simulink model "Resp18e_updatedPulse"  (Simulink 7.3)
settings: Solver=ode23  StartTime=0.0  StopTime=20  FixedStep=0.01  MaxStep=0.05  RelTol=1e-6
values from neighbouring files (symbols this model uses):
  alpha_CO2_brain = 2.9/1e3*760/P_stp/K_stp    (= 0.00097047576489)    [initialize_parameters.m]
  alpha_CO2_fat = 0.9/K_stp/P_stp    (= 0.000396292281489)    [initialize_parameters.m]
  alpha_CO2_heart = 2.4/1e3*760/P_stp/K_stp    (= 0.00080315235715)    [initialize_parameters.m]
  alpha_CO2_lean = 4.2/1e3*760/P_stp/K_stp    (= 0.00140551662501)    [initialize_parameters.m]
  alpha_CO2_lungtiss_fast = alpha_CO2_lungtiss_fast./0.1333    [initialize_parameters.m]
  alpha_CO2_muscle = 4.2/1e3*760/P_stp/K_stp    (= 0.00140551662501)    [initialize_parameters.m]
  alpha_CO2_other = 3.0/1e3*760/P_stp/K_stp    (= 0.00100394044644)    [initialize_parameters.m]
  alpha_O2_fat = 5*0.024/K_stp/P_stp    (= 5.28389708651e-05)    [initialize_parameters.m]
  alpha_O2_tissue = 0.024/K_stp/P_stp    (= 1.0567794173e-05)    [initialize_parameters.m]
  BOHRF0 = O2_SHIFT - T_BLOOD_M_37 * (0.024 + BOHRF * 0.0147) - BOHRF1 * 7.4    (= -3.552)    [initialize_parameters.m]
  BOHRF1 = BOHRF * (1 - T_BLOOD_M_37 * 0.0065)    (= 0.48)    [initialize_parameters.m]
  C_a_CO2_i = 20.8e-3    (= 0.0208)    [initialize_parameters.m]    (also in resp18e_ic_norm.mat = 0.0202734801806)
  C_a_O2_i = 8.95e-3    (= 0.00895)    [initialize_parameters.m]    (also in resp18e_ic_norm.mat = 0.00918087581167)
  CAP_O2 = 0.01 * CAP_O2    (= 0.201)    [initialize_parameters.m]
  Cardiac_duty_cycle = 40    [initialize_parameters.m]
  Co_CO2_brain = 401*K_Co_CO2/1e3/K_stp    (= 0.0107345869894)    [initialize_parameters.m]
  Co_CO2_heart = 487*K_Co_CO2/1e3/K_stp    (= 0.0130367677403)    [initialize_parameters.m]
  Co_CO2_lean = 342*K_Co_CO2/1e3/K_stp    (= 0.00915518391618)    [initialize_parameters.m]
  Co_CO2_muscle = 342*K_Co_CO2/1e3/K_stp    (= 0.00915518391618)    [initialize_parameters.m]
  Co_CO2_other = 355*K_Co_CO2/1e3/K_stp    (= 0.00950318798317)    [initialize_parameters.m]
  DH2ODS = DH2ODS + 0.007 * HB_MEQ * (HB_MEQ - 9) / (13.5 * (13.5 - 9))    (= 0.00498709726946)    [initialize_parameters.m]
  F_insp_alv_alvds = F_v_alv_deadspace / F_insp_hivq    (= 0.00299401197605)    [initialize_parameters.m]
  F_insp_alv_hivq = F_v_alv_hivq      / F_insp_hivq    (= 0.997005988024)    [initialize_parameters.m]
  F_insp_alv_lovq = F_v_alv_lovq      / F_insp_lovq    (= 0.5)    [initialize_parameters.m]
  F_insp_alv_midvq = F_v_alv_midvq     / F_insp_lovq    (= 0.5)    [initialize_parameters.m]
  F_insp_hivq = F_v_alv_deadspace + F_v_alv_hivq    (= 0.334)    [initialize_parameters.m]
  F_insp_lovq = F_v_alv_midvq     + F_v_alv_lovq    (= 0.666)    [initialize_parameters.m]
  Fi_CO2_param_est = 0.01    [initialize_parameters.m]
  Fi_error = 1e-6    (= 1e-06)    [initialize_parameters.m]
  Fi_N2_mean = 1-(Fi_O2_mean + Fi_N2O_mean)    (= 0.65)    [initialize_parameters.m]
  Fi_O2_mean = 0.35    [initialize_parameters.m]
  Fi_O2_param_est = 0.01    [initialize_parameters.m]
  Fq_brain = 0.114    [initialize_parameters.m]
  Fq_error = 1e-8    (= 1e-08)    [initialize_parameters.m]
  Fq_fat = 0.103    [initialize_parameters.m]
  Fq_heart = 0.041    [initialize_parameters.m]
  Fq_hepatic = 0.069    [initialize_parameters.m]
  Fq_kidneys = 0.215    [initialize_parameters.m]
  Fq_lean = 0.090    (= 0.09)    [initialize_parameters.m]
  Fq_lungs_anatomicalshunt = 0.01    [initialize_parameters.m]
  Fq_lungs_hivq = (1-Fq_lungs_pulmshunt-Fq_lungs_anatomicalshunt)    *F_v_alv_hivq/(F_v_alv_hivq+F_v_alv_midvq+F_v_alv_lovq)    (= 0.3)    [initialize_parameters.m]
  Fq_lungs_lovq = (1-Fq_lungs_pulmshunt-Fq_lungs_anatomicalshunt)    *F_v_alv_lovq/(F_v_alv_hivq+F_v_alv_midvq+F_v_alv_lovq)    (= 0.3)    [initialize_parameters.m]
  Fq_lungs_midvq = (1-Fq_lungs_pulmshunt-Fq_lungs_anatomicalshunt)    *F_v_alv_midvq/(F_v_alv_hivq+F_v_alv_midvq+F_v_alv_lovq)    (= 0.3)    [initialize_parameters.m]
  Fq_lungs_pulmshunt = 0.09    [initialize_parameters.m]
  Fq_muscle = 0.096    [initialize_parameters.m]
  Fq_pershunt = 0.101    [initialize_parameters.m]
  Fq_portal = 0.171    [initialize_parameters.m]
  FRC = 2.2    [initialize_parameters.m]
  H2OB = H2OVC + 0.938 * (1 - VC_74)    (= 0.840191964286)    [initialize_parameters.m]
  k_CO2_lungtiss_fast_alvds = k_CO2_lungtiss_fast*F_v_alv_deadspace    (= 3.63090772693e-07)    [initialize_parameters.m]
  k_CO2_lungtiss_fast_hivq = k_CO2_lungtiss_fast*F_v_alv_hivq    (= 0.000120909227307)    [initialize_parameters.m]
  k_CO2_lungtiss_fast_lovq = k_CO2_lungtiss_fast*F_v_alv_lovq    (= 0.000120909227307)    [initialize_parameters.m]
  k_CO2_lungtiss_fast_midvq = k_CO2_lungtiss_fast*F_v_alv_midvq    (= 0.000120909227307)    [initialize_parameters.m]
  k_CO2_lungtiss_slow_alvds = k_CO2_lungtiss_slow*F_v_alv_deadspace    (= 4.95123780945e-09)    [initialize_parameters.m]
  k_CO2_lungtiss_slow_hivq = k_CO2_lungtiss_slow*F_v_alv_hivq    (= 1.64876219055e-06)    [initialize_parameters.m]
  k_CO2_lungtiss_slow_lovq = k_CO2_lungtiss_slow*F_v_alv_lovq    (= 1.64876219055e-06)    [initialize_parameters.m]
  k_CO2_lungtiss_slow_midvq = k_CO2_lungtiss_slow*F_v_alv_midvq    (= 1.64876219055e-06)    [initialize_parameters.m]
  K_diff_CO2_hivq = K_diff_CO2*F_v_alv_hivq    (= 0.0014985)    [initialize_parameters.m]
  K_diff_CO2_lovq = K_diff_CO2*F_v_alv_lovq    (= 0.0014985)    [initialize_parameters.m]
  K_diff_CO2_midvq = K_diff_CO2*F_v_alv_midvq    (= 0.0014985)    [initialize_parameters.m]
  K_diff_O2_hivq = K_diff_O2*F_v_alv_hivq    (= 7.326e-05)    [initialize_parameters.m]
  K_diff_O2_lovq = K_diff_O2*F_v_alv_lovq    (= 7.326e-05)    [initialize_parameters.m]
  K_diff_O2_midvq = K_diff_O2*F_v_alv_midvq    (= 7.326e-05)    [initialize_parameters.m]
  K_exp_alv_alvds = 1/1    (= 1)    [initialize_parameters.m]
  K_exp_alv_hivq = 1/1    (= 1)    [initialize_parameters.m]
  K_press = 760/101.325    (= 7.50061682704)    [initialize_parameters.m]
  K_stp = R*(T_stp+273.15)/(P_stp*1000)    (= 22.4135311621)    [initialize_parameters.m]
  Kg_alv = R*(T_alv+273.15)/(P_baro*1000)    (= 25.3668469802)    [initialize_parameters.m]
  LN10 = 2.30258509299405    (= 2.30258509299)    [initialize_parameters.m]
  m_alv_alvds_i = (FRC-V_deadspace_total)/Kg_alv * F_v_alv_deadspace    [initialize_parameters.m]
  m_alv_hivq_i = (FRC-V_deadspace_total)/Kg_alv * F_v_alv_hivq    [initialize_parameters.m]
  m_alv_lovq_i = (FRC-V_deadspace_total)/Kg_alv * F_v_alv_lovq    [initialize_parameters.m]
  m_alv_midvq_i = (FRC-V_deadspace_total)/Kg_alv * F_v_alv_midvq    [initialize_parameters.m]
  m_CO2_alv_alvds_i = F_CO2_i * m_alv_alvds_i    [initialize_parameters.m]
  m_CO2_alv_hivq_i = F_CO2_i * m_alv_hivq_i    [initialize_parameters.m]
  m_CO2_alv_lovq_i = F_CO2_i * m_alv_lovq_i    [initialize_parameters.m]
  m_CO2_alv_midvq_i = F_CO2_i * m_alv_midvq_i    [initialize_parameters.m]
  m_CO2_brain_b_i = C_a_CO2_i*Vb_brain    (= 0.002184)    [initialize_parameters.m]
  m_CO2_brain_t_i = (Co_CO2_brain  + alpha_CO2_brain *P_v_CO2_i)* Vt_brain    (= 0.0171268217946)    [initialize_parameters.m]
  m_CO2_common_b_i = C_a_CO2_i*Vb_common    (= 0.0170421333333)    [initialize_parameters.m]
  m_CO2_ds0_i = F_CO2_i*m_ds0_i    (= 0.000985538329597)    [initialize_parameters.m]
  m_CO2_ds_large_i = F_CO2_i * m_deadspace_large_1    [initialize_parameters.m]
  m_CO2_ds_med_hivq1_i = F_CO2_i * m_deadspace_med_hivq_1    [initialize_parameters.m]
  m_CO2_ds_med_hivq2_i = F_CO2_i * m_deadspace_med_hivq_2    [initialize_parameters.m]
  m_CO2_ds_med_lovq1_i = F_CO2_i * m_deadspace_med_lovq_1    [initialize_parameters.m]
  m_CO2_ds_med_lovq2_i = F_CO2_i * m_deadspace_med_lovq_2    [initialize_parameters.m]
  m_CO2_ds_small_alvds_i = F_CO2_i * m_deadspace_small_alvdeadspace    [initialize_parameters.m]
  m_CO2_ds_small_hivq_i = F_CO2_i * m_deadspace_small_hivq    [initialize_parameters.m]
  m_CO2_ds_small_lovq_i = F_CO2_i * m_deadspace_small_lovq    [initialize_parameters.m]
  m_CO2_ds_small_midvq_i = F_CO2_i * m_deadspace_small_midvq    [initialize_parameters.m]
  m_CO2_fat_b_i = C_a_CO2_i*Vb_fat    (= 0.0116896)    [initialize_parameters.m]
  m_CO2_fat_t_i = P_a_CO2_i*alpha_CO2_fat*Vt_fat    (= 0.0302752719501)    [initialize_parameters.m]
  m_CO2_heart_b_i = C_a_CO2_i*Vb_heart    (= 0.000832)    [initialize_parameters.m]
  m_CO2_heart_t_i = (Co_CO2_heart  + alpha_CO2_heart *P_v_CO2_i)* Vt_heart    (= 0.00402544335149)    [initialize_parameters.m]
  m_CO2_hepatic_b_i = C_a_CO2_i*Vb_hepatic    (= 0.0019136)    [initialize_parameters.m]
  m_CO2_kidneys_b_i = C_a_CO2_i*Vb_kidneys    (= 0.0012064)    [initialize_parameters.m]
  m_CO2_kidneys_t_i = (Co_CO2_other  + alpha_CO2_other *P_v_CO2_i)* Vt_kidneys    (= 0.0045902552907)    [initialize_parameters.m]
  m_CO2_lean_b_i = C_a_CO2_i*Vb_lean    (= 0.0191984)    [initialize_parameters.m]
  m_CO2_lean_t_i = (Co_CO2_lean   + alpha_CO2_lean  *P_v_CO2_i)* Vt_lean    (= 0.0884995401953)    [initialize_parameters.m]
  m_CO2_liver_t_i = (Co_CO2_other  + alpha_CO2_other *P_v_CO2_i)* Vt_liver    (= 0.0187019339777)    [initialize_parameters.m]
  m_CO2_lungtiss_fast_alvds_i = F_CO2_i*(P_baro-P_A_H2O)*V_lungtiss_alvds *alpha_CO2_lungtiss_fast(2)    [initialize_parameters.m]
  m_CO2_lungtiss_fast_hivq_i = F_CO2_i*(P_baro-P_A_H2O)*V_lungtiss_hivq  *alpha_CO2_lungtiss_fast(2)    [initialize_parameters.m]
  m_CO2_lungtiss_fast_lovq_i = F_CO2_i*(P_baro-P_A_H2O)*V_lungtiss_lovq  *alpha_CO2_lungtiss_fast(2)    [initialize_parameters.m]
  m_CO2_lungtiss_fast_midvq_i = F_CO2_i*(P_baro-P_A_H2O)*V_lungtiss_midvq *alpha_CO2_lungtiss_fast(2)    [initialize_parameters.m]
  m_CO2_lungtiss_slow_alvds_i = F_CO2_i*(P_baro-P_A_H2O)*V_lungtiss_alvds*alpha_CO2_lungtiss_slow    [initialize_parameters.m]
  m_CO2_lungtiss_slow_hivq_i = F_CO2_i*(P_baro-P_A_H2O)*V_lungtiss_hivq *alpha_CO2_lungtiss_slow    [initialize_parameters.m]
  m_CO2_lungtiss_slow_lovq_i = F_CO2_i*(P_baro-P_A_H2O)*V_lungtiss_lovq *alpha_CO2_lungtiss_slow    [initialize_parameters.m]
  m_CO2_lungtiss_slow_midvq_i = F_CO2_i*(P_baro-P_A_H2O)*V_lungtiss_midvq*alpha_CO2_lungtiss_slow    [initialize_parameters.m]
  m_CO2_LV_b_i = C_a_CO2_i*Vb_LV    (= 0.00391733333333)    [initialize_parameters.m]
  m_CO2_muscle_b_i = C_a_CO2_i*Vb_muscle    (= 0.0201344)    [initialize_parameters.m]
  m_CO2_muscle_t_i = (Co_CO2_muscle + alpha_CO2_muscle*P_v_CO2_i)* Vt_muscle    (= 0.363660431061)    [initialize_parameters.m]
  m_CO2_pershunt_b_i = C_a_CO2_i*Vb_pershunt    (= 0.0027248)    [initialize_parameters.m]
  m_CO2_portal_b_i = C_a_CO2_i*Vb_portal    (= 0.0210912)    [initialize_parameters.m]
  m_CO2_portal_t_i = (Co_CO2_other  + alpha_CO2_other *P_v_CO2_i)* Vt_portal    (= 0.0164739329706)    [initialize_parameters.m]
  m_CO2_pulmcap_b_hivq_i = C_a_CO2_i*Vb_pulmcap_hivq    (= 0.000630933333333)    [initialize_parameters.m]
  m_CO2_pulmcap_b_lovq_i = C_a_CO2_i*Vb_pulmcap_lovq    (= 0.000630933333333)    [initialize_parameters.m]
  m_CO2_pulmcap_b_midvq_i = C_a_CO2_i*Vb_pulmcap_midvq    (= 0.000630933333333)    [initialize_parameters.m]
  m_CO2_pulmcap_b_pulmshunt_i = C_a_CO2_i*Vb_pulmcap_pulmshunt    (= 0.0001872)    [initialize_parameters.m]
  m_CO2_RV_b_i = C_v_CO2_i*Vb_RV    (= 0.004181)    [initialize_parameters.m]
  m_N2_alv_alvds_i = Fi_N2_mean * (m_alv_alvds_i - m_CO2_alv_alvds_i)    [initialize_parameters.m]
  ... (+122 more)
undefined symbols (not defined in the file or in its folder): AH2OVC, AHCO3B, DHCO3BDS, litres, mole
libraries: simulink x28
(part 1 of 8)
settings Model: Creator=MJTurner  LastModifiedBy=John  ExtModeTrigMode=oneshot  ExtModeArmWhenConnect=off
settings SolverCC: InitialStep=0.0001  MaxOrder=3
settings DataIOCC: FinalStateName=x_final  InitialState=x_initial  LimitDataPoints=off  LoadInitialState=on  SaveFinalState=on  SaveOutput=off  StateSaveName=x_states  TimeSaveName=t
settings OptimizationCC: BlockReduction=off  BooleanDataType=off  InitFltsAndDblsToZero=on
settings DebuggingCC: AlgebraicLoopMsg=none  SaveWithParameterizedLinksMsg=none  SignalResolutionControl=TryResolveAllWithWarning  SolverPrmCheckMsg=none  MultiTaskDSMMsg=warning  MultiTaskCondExecSysMsg=none  StrictBusMsg=None
settings HardwareCC: TargetUnknown=on
settings RTWCC: TemplateMakefile=grt_vc.tmf  IncludeERTFirstTime=on
settings GRTTargetCC: TargetFcnLib=ansi_tfl_tmw.mat

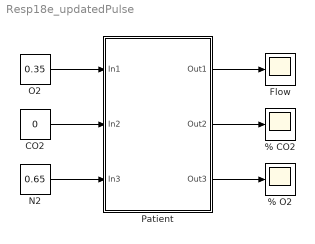
== system Resp18e_updatedPulse ==
  % CO2 : Scope
      settings: YMin=0  YMax=5.25  SaveName=ScopeData9
  % O2 : Scope
      settings: YMin=28.5  YMax=35  SaveName=ScopeData8
  CO2 : Constant  Value=0  OutDataType=fixdt(1, 16)  OutScaling=2^0
  Flow : Scope
      settings: YMin=-0.02  YMax=0.0175  SaveName=ScopeData10
  N2 : Constant  Value=0.65  OutDataType=fixdt(1, 16)  OutScaling=2^0
  O2 : Constant  Value=0.35  OutDataType=fixdt(1, 16)  OutScaling=2^0
  Patient : Subsystem
  wires:
  O2/1 -> Patient/1(In1)
  CO2/1 -> Patient/2(In2)
  N2/1 -> Patient/3(In3)
  Patient/3(Out3) -> % O2/1
  Patient/1(Out1) -> Flow/1
  Patient/2(Out2) -> % CO2/1

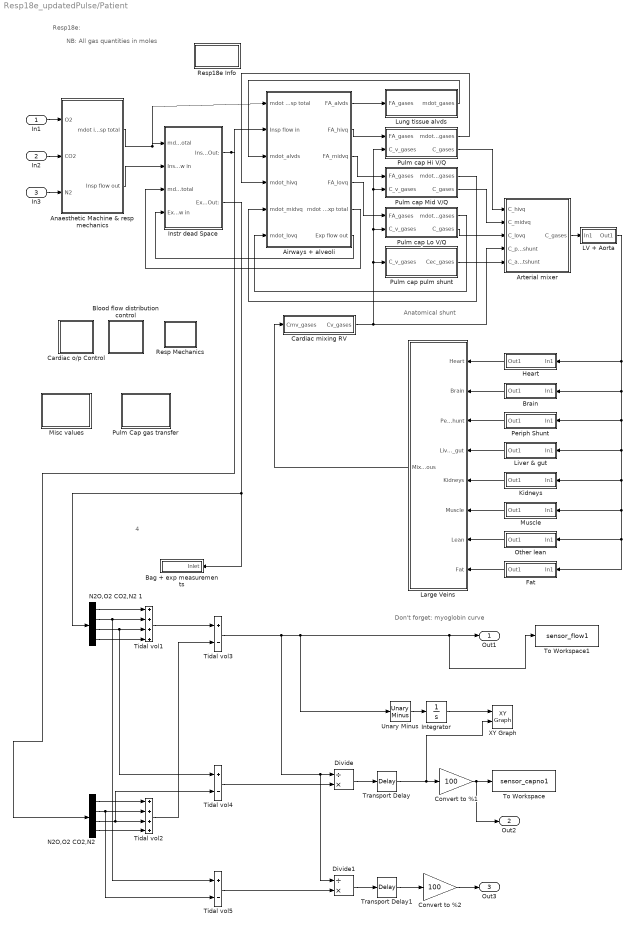
== system Resp18e_updatedPulse/Patient ==
  note: Resp18e:
  note: NB: All gas quantities in moles
  note: Anatomical shunt
  note: 4
  note: Don't forget: myoglobin curve
  In1 : Inport
  In2 : Inport  Port=2
  In3 : Inport  Port=3
  Airways + alveoli : Subsystem
  Anaesthetic Machine & resp mechanics : Subsystem
  Arterial mixer : Subsystem
  Bag + exp measurements : Subsystem
  Blood flow distribution control : Subsystem
  Brain : Subsystem
  Cardiac mixing RV : Subsystem
  Cardiac o/p Control : Subsystem
  Convert to %1 : Gain  Gain=100  ParameterDataType=fixdt(1, 16)  ParameterScaling=2^0  OutDataType=fixdt(1, 16)  OutScaling=2^0
  Convert to %2 : Gain  Gain=100  ParameterDataType=fixdt(1, 16)  ParameterScaling=2^0  OutDataType=fixdt(1, 16)  OutScaling=2^0
  Divide : Product  Inputs=/*  OutDataType=fixdt(1, 16)  OutScaling=2^-10
  Divide1 : Product  Inputs=/*  OutDataType=fixdt(1, 16)  OutScaling=2^-10
  Fat : Subsystem
  Heart : Subsystem
  Instr dead Space : Subsystem
  Integrator : Integrator  ZeroCross=off  ContinuousStateAttributes='volumeIntegrator'
  Kidneys : Subsystem
  LV + Aorta : Subsystem
  Large Veins : Subsystem
  Liver & gut : Subsystem
  Lung tissue alvds : Subsystem
  Misc values : Subsystem
  Muscle : Subsystem
  "N2O,O2 CO2,N2 " : Demux
  N2O,O2 CO2,N2 1 : Demux
  Other lean : Subsystem
  Periph Shunt : Subsystem
  Pulm Cap gas transfer : Subsystem
  Pulm cap Hi V/Q : Subsystem
  Pulm cap Lo V/Q : Subsystem
  Pulm cap Mid V/Q : Subsystem
  Pulm cap pulm shunt : Subsystem
  Resp Mechanics : Subsystem
  Resp18e Info : Subsystem
  Tidal vol1 : Sum  Inputs=++++  OutDataType=sfix(16)  OutScaling=2^0  SaturateOnIntegerOverflow=on  InputSameDT=on  OutDataTypeStr=Inherit: Same as first input
  Tidal vol2 : Sum  Inputs=++++  OutDataType=sfix(16)  OutScaling=2^0  SaturateOnIntegerOverflow=on  InputSameDT=on  OutDataTypeStr=Inherit: Same as first input
  Tidal vol3 : Sum  Inputs=+-  OutDataType=sfix(16)  OutScaling=2^0  SaturateOnIntegerOverflow=on  InputSameDT=on  OutDataTypeStr=Inherit: Same as first input
  Tidal vol4 : Sum  Inputs=+-  OutDataType=sfix(16)  OutScaling=2^0  SaturateOnIntegerOverflow=on  InputSameDT=on  OutDataTypeStr=Inherit: Same as first input
  Tidal vol5 : Sum  Inputs=+-  OutDataType=sfix(16)  OutScaling=2^0  SaturateOnIntegerOverflow=on  InputSameDT=on  OutDataTypeStr=Inherit: Same as first input
  To Workspace : ToWorkspace  VariableName=sensor_capno1  SampleTime=t_sample_sensor  SaveFormat=Array
  To Workspace1 : ToWorkspace  VariableName=sensor_flow1  SampleTime=t_sample_sensor  SaveFormat=Array
  Transport Delay : TransportDelay  DelayTime=0.01
  Transport Delay1 : TransportDelay  DelayTime=0.01
  Unary Minus : simulink/Math Operations/Unary Minus  DoSatur=off
  XY Graph : simulink/Sinks/XY Graph  SystemSampleTime=-1  xmin=-0.05  xmax=0.05  ymin=0  ymax=0.08  st=-1
  Out1 : Outport
  Out2 : Outport  Port=2
  Out3 : Outport  Port=3
  wires:
  Anaesthetic Machine & resp mechanics/2(Insp flow out) -> Instr dead Space/2(Insp flow in)
  Instr dead Space/2(Exp flow Out:) -> Bag + exp measurements/1(Inlet), N2O,O2 CO2,N2 1/1
  Anaesthetic Machine & resp mechanics/1(mdot insp total) -> Instr dead Space/1(mdot InspTotal), Airways + alveoli/1(mdot insp total)
  Instr dead Space/1(Insp flow Out:) -> Airways + alveoli/2(Insp flow in), "N2O,O2 CO2,N2 "/1
  Airways + alveoli/6(Exp flow out) -> Instr dead Space/4(Exp flow in)
  Arterial mixer/1(C_gases) -> LV + Aorta/1(In1)
  Airways + alveoli/2(FA_hivq) -> Pulm cap Hi V/Q/1(FA_gases)
  Airways + alveoli/3(FA_midvq) -> Pulm cap Mid V/Q/1(FA_gases)
  Airways + alveoli/4(FA_lovq) -> Pulm cap Lo V/Q/1(FA_gases)
  Pulm cap Lo V/Q/1(mdot_gases) -> Airways + alveoli/6(mdot_lovq)
  Pulm cap Mid V/Q/1(mdot_gases) -> Airways + alveoli/5(mdot_midvq)
  Pulm cap Hi V/Q/1(mdot_gases) -> Airways + alveoli/4(mdot_hivq)
  Pulm cap Lo V/Q/2(C_gases) -> Arterial mixer/3(C_lovq)
  Pulm cap Mid V/Q/2(C_gases) -> Arterial mixer/2(C_midvq)
  Pulm cap Hi V/Q/2(C_gases) -> Arterial mixer/1(C_hivq)
  Lung tissue alvds/1(mdot_gases) -> Airways + alveoli/3(mdot_alvds)
  Airways + alveoli/1(FA_alvds) -> Lung tissue alvds/1(FA_gases)
  Liver & gut/1(Out1) -> Large Veins/4(Liver_gut)
  LV + Aorta/1(Out1) -> Heart/1(In1), Liver & gut/1(In1), Kidneys/1(In1), Muscle/1(In1), Other lean/1(In1), Fat/1(In1), Periph Shunt/1(In1), Brain/1(In1)
  Heart/1(Out1) -> Large Veins/1(Heart)
  Kidneys/1(Out1) -> Large Veins/5(Kidneys)
  Muscle/1(Out1) -> Large Veins/6(Muscle)
  Other lean/1(Out1) -> Large Veins/7(Lean)
  Fat/1(Out1) -> Large Veins/8(Fat)
  Brain/1(Out1) -> Large Veins/2(Brain)
  Periph Shunt/1(Out1) -> Large Veins/3(Per shunt)
  Cardiac mixing RV/1(Cv_gases) -> Arterial mixer/4(C_pulmshunt), Pulm cap Lo V/Q/2(C_v_gases), Pulm cap Mid V/Q/2(C_v_gases), Pulm cap Hi V/Q/2(C_v_gases), Pulm cap pulm shunt/1(C_v_gases)
  Large Veins/1(Mixed Venous) -> Cardiac mixing RV/1(Cmv_gases)
  Pulm cap pulm shunt/1(Cec_gases) -> Arterial mixer/5(C_anatshunt)
  Airways + alveoli/5(mdot exp total) -> Instr dead Space/3(mdot exp total)
  N2O,O2 CO2,N2 1/1 -> Tidal vol1/1
  N2O,O2 CO2,N2 1/4 -> Tidal vol1/4
  N2O,O2 CO2,N2 1/2 -> Tidal vol1/2, Tidal vol5/1
  "N2O,O2 CO2,N2 "/1 -> Tidal vol2/1
  "N2O,O2 CO2,N2 "/2 -> Tidal vol2/2, Tidal vol5/2
  Tidal vol1/1 -> Tidal vol3/1
  N2O,O2 CO2,N2 1/3 -> Tidal vol1/3, Tidal vol4/1
  "N2O,O2 CO2,N2 "/3 -> Tidal vol2/3, Tidal vol4/2
  "N2O,O2 CO2,N2 "/4 -> Tidal vol2/4
  Tidal vol2/1 -> Tidal vol3/2
  Tidal vol4/1 -> Divide/2
  Tidal vol3/1 -> Unary Minus/1, To Workspace1/1, Out1/1, Divide/1, Divide1/1
  Divide/1 -> Transport Delay/1
  Transport Delay/1 -> XY Graph/2, Convert to %1/1
  Integrator/1 -> XY Graph/1
  Unary Minus/1 -> Integrator/1
  Divide1/1 -> Transport Delay1/1
  Tidal vol5/1 -> Divide1/2
  In1/1 -> Anaesthetic Machine & resp mechanics/1(O2)
  In2/1 -> Anaesthetic Machine & resp mechanics/2(CO2)
  In3/1 -> Anaesthetic Machine & resp mechanics/3(N2)
  Transport Delay1/1 -> Convert to %2/1
  Convert to %1/1 -> To Workspace/1, Out2/1
  Convert to %2/1 -> Out3/1

== system Resp18e_updatedPulse/Patient/Airways + alveoli ==
  note: This subsystem has multiple lung compartments
      | See Weibel Model 'A' Regular dichotomy page 136
  note: Large airways
      | Weibel generations 0 - 5
      | total nominal vol: 50.4 ml
      | N=1 - 8
      | Convective transport dominates
  note: Medium airways
      | Weibel generations 6 - 17
      | N = 16 - 131 000
  note: Small airways
      | Weibel generations 18 - 20
      | N = 262 000 - 524 000
      | Diffusion dominant
  note: Weibel generations 21 - 23
      | + alveolar vol
  mdot insp total : Inport  OutDataType=sfix(16)  OutScaling=2^0
  Insp flow in : Inport  Port=2  OutDataType=sfix(16)  OutScaling=2^0
  mdot_alvds : Inport  Port=3  OutDataType=sfix(16)  OutScaling=2^0
  mdot_hivq : Inport  Port=4  OutDataType=sfix(16)  OutScaling=2^0
  mdot_midvq : Inport  Port=5  OutDataType=sfix(16)  OutScaling=2^0
  mdot_lovq : Inport  Port=6  OutDataType=sfix(16)  OutScaling=2^0
  Alv compartment alvds : Subsystem  Description=ALveolar compartment
  Alv compartment hi V/Q : Subsystem  Description=ALveolar compartment
  Alv compartment lo V/Q : Subsystem  Description=ALveolar compartment
  Alv compartment mid V/Q : Subsystem  Description=ALveolar compartment
  F_1_2_1 : Gain  Gain=F_insp_hivq  ParameterDataType=sfix(16)  ParameterScaling=2^0  OutDataType=sfix(16)  OutScaling=2^0  SaturateOnIntegerOverflow=on  OutDataTypeStr=Inherit: Same as input  ParamDataTypeStr=Inherit: Same as input
  F_1_2_2 : Gain  Gain=F_insp_lovq  ParameterDataType=sfix(16)  ParameterScaling=2^0  OutDataType=sfix(16)  OutScaling=2^0  SaturateOnIntegerOverflow=on  OutDataTypeStr=Inherit: Same as input  ParamDataTypeStr=Inherit: Same as input
  F_2_3_b : Gain  Gain=F_insp_alv_hivq  ParameterDataType=sfix(16)  ParameterScaling=2^0  OutDataType=sfix(16)  OutScaling=2^0  SaturateOnIntegerOverflow=on  OutDataTypeStr=Inherit: Same as input  ParamDataTypeStr=Inherit: Same as input
  F_2_3a : Gain  Gain=F_insp_alv_alvds  ParameterDataType=sfix(16)  ParameterScaling=2^0  OutDataType=sfix(16)  OutScaling=2^0  SaturateOnIntegerOverflow=on  OutDataTypeStr=Inherit: Same as input  ParamDataTypeStr=Inherit: Same as input
  F_2_3c : Gain  Gain=F_insp_alv_midvq  ParameterDataType=sfix(16)  ParameterScaling=2^0  OutDataType=sfix(16)  OutScaling=2^0  SaturateOnIntegerOverflow=on  OutDataTypeStr=Inherit: Same as input  ParamDataTypeStr=Inherit: Same as input
  F_2_3d : Gain  Gain=F_insp_alv_lovq  ParameterDataType=sfix(16)  ParameterScaling=2^0  OutDataType=sfix(16)  OutScaling=2^0  SaturateOnIntegerOverflow=on  OutDataTypeStr=Inherit: Same as input  ParamDataTypeStr=Inherit: Same as input
  Series dead Space alv dead sp : Subsystem
  Series dead Space hi V/Q : Subsystem
  Series dead Space lo V/Q : Subsystem
  Series dead Space mid V/Q : Subsystem
  Series deadspace large_1 : Subsystem
  Series deadspace large_2 : Subsystem
  Series deadspace large_3 : Subsystem
  Series deadspace medium HiVQ 2 : Subsystem
  Series deadspace medium hiVQ 1 : Subsystem
  Series deadspace medium med_lo VQ 1 : Subsystem
  Series deadspace medium med_loVQ 2 : Subsystem
  Sum : Sum  OutDataType=sfix(16)  OutScaling=2^0  SaturateOnIntegerOverflow=on  InputSameDT=on  OutDataTypeStr=Inherit: Same as first input
  Sum1 : Sum  OutDataType=sfix(16)  OutScaling=2^0  SaturateOnIntegerOverflow=on  InputSameDT=on  OutDataTypeStr=Inherit: Same as first input
  Sum2 : Sum  OutDataType=sfix(16)  OutScaling=2^0  SaturateOnIntegerOverflow=on  InputSameDT=on  OutDataTypeStr=Inherit: Same as first input
  FA_alvds : Outport  OutDataType=sfix(16)  OutScaling=2^0
  FA_hivq : Outport  Port=2  OutDataType=sfix(16)  OutScaling=2^0
  FA_midvq : Outport  Port=3  OutDataType=sfix(16)  OutScaling=2^0
  FA_lovq : Outport  Port=4  OutDataType=sfix(16)  OutScaling=2^0
  mdot exp total : Outport  Port=5  OutDataType=sfix(16)  OutScaling=2^0
  Exp flow out : Outport  Port=6  OutDataType=sfix(16)  OutScaling=2^0
  wires:
  Series deadspace large_1/1(Insp flow  Out:) -> Series deadspace large_2/2(Insp flow in)
  mdot insp total/1 -> Series deadspace large_1/1(mdot insp total), Series deadspace large_2/1(mdot insp total), Series deadspace large_3/1(mdot insp total)
  Insp flow in/1 -> Series deadspace large_1/2(Insp flow in)
  Series deadspace large_2/2(Exp flow  Out:) -> Series deadspace large_1/4(Exp flow in)
  F_2_3_b/1 -> Series dead Space hi V/Q/1(Insp flow in)
  F_2_3d/1 -> Series dead Space lo V/Q/1(Insp flow in)
  F_2_3c/1 -> Series dead Space mid V/Q/1(Insp flow in)
  Series dead Space hi V/Q/2(Exp flow  Out:) -> Sum1/2
  Sum1/1 -> Series deadspace medium HiVQ 2/2(Exp flow in)
  Sum2/1 -> Series deadspace medium med_loVQ 2/2(Exp flow in)
  Series dead Space mid V/Q/2(Exp flow  Out:) -> Sum2/1
  Series dead Space lo V/Q/2(Exp flow  Out:) -> Sum2/2
  F_1_2_1/1 -> Series deadspace medium hiVQ 1/1(Insp flow in)
  Series deadspace medium hiVQ 1/1(Insp flow  Out:) -> Series deadspace medium HiVQ 2/1(Insp flow in)
  Series deadspace medium HiVQ 2/2(Exp flow  Out:) -> Series deadspace medium hiVQ 1/2(Exp flow in)
  Series deadspace medium hiVQ 1/2(Exp flow  Out:) -> Sum/1
  F_1_2_2/1 -> Series deadspace medium med_lo VQ 1/1(Insp flow in)
  Series deadspace medium med_lo VQ 1/1(Insp flow  Out:) -> Series deadspace medium med_loVQ 2/1(Insp flow in)
  Series deadspace medium med_loVQ 2/2(Exp flow  Out:) -> Series deadspace medium med_lo VQ 1/2(Exp flow in)
  Series deadspace medium med_lo VQ 1/2(Exp flow  Out:) -> Sum/2
  Series deadspace medium HiVQ 2/1(Insp flow  Out:) -> F_2_3a/1, F_2_3_b/1
  Series deadspace medium med_loVQ 2/1(Insp flow  Out:) -> F_2_3c/1, F_2_3d/1
  Series dead Space hi V/Q/1(Insp flow  Out:) -> Alv compartment hi V/Q/1(Insp flow in)
  Series dead Space lo V/Q/1(Insp flow  Out:) -> Alv compartment lo V/Q/1(Insp flow in)
  Series dead Space mid V/Q/1(Insp flow  Out:) -> Alv compartment mid V/Q/1(Insp flow in)
  Alv compartment hi V/Q/1(Exp flow  Out:) -> Series dead Space hi V/Q/2(Exp flow in)
  Alv compartment mid V/Q/1(Exp flow  Out:) -> Series dead Space mid V/Q/2(Exp flow in)
  Alv compartment lo V/Q/1(Exp flow  Out:) -> Series dead Space lo V/Q/2(Exp flow in)
  Alv compartment hi V/Q/2(FA_gases) -> FA_hivq/1
  mdot_hivq/1 -> Alv compartment hi V/Q/2(mdot_gases)
  mdot_midvq/1 -> Alv compartment mid V/Q/2(mdot_gases)
  Alv compartment mid V/Q/2(FA_gases) -> FA_midvq/1
  mdot_lovq/1 -> Alv compartment lo V/Q/2(mdot_gases)
  Alv compartment lo V/Q/2(FA_gases) -> FA_lovq/1
  Series deadspace large_3/1(Insp flow  Out:) -> F_1_2_1/1, F_1_2_2/1
  Series deadspace large_2/1(Insp flow  Out:) -> Series deadspace large_3/2(Insp flow in)
  Sum/1 -> Series deadspace large_3/3(Exp flow in)
  Series deadspace large_3/2(Exp flow  Out:) -> Series deadspace large_2/4(Exp flow in)
  Series deadspace large_1/2(Exp flow  Out:) -> Exp flow out/1
  F_2_3a/1 -> Series dead Space alv dead sp/1(Insp flow in)
  Series dead Space alv dead sp/2(Exp flow  Out:) -> Sum1/1
  Series dead Space alv dead sp/1(Insp flow  Out:) -> Alv compartment alvds/1(Insp flow in)
  mdot_alvds/1 -> Alv compartment alvds/2(mdot_gases)
  Alv compartment alvds/2(FA_gases) -> FA_alvds/1
  Alv compartment alvds/1(Exp flow  Out:) -> Series dead Space alv dead sp/2(Exp flow in)
  Series deadspace large_3/3(mdot exp total) -> Series deadspace large_1/3(mdot exp Total), Series deadspace large_2/3(mdot exp total), mdot exp total/1

== system Resp18e_updatedPulse/Patient/Anaesthetic Machine & resp mechanics ==
  note: Anaesthetic machine & resp mechanics
  note: 4th gas (N2O or H2O) unused
  note: N2O
      | O2
      | CO2
      | N2
  O2 : Inport  OutDataType=fixdt(1, 16)  OutScaling=2^0
  CO2 : Inport  Port=2  OutDataType=fixdt(1, 16)  OutScaling=2^0
  N2 : Inport  Port=3  OutDataType=fixdt(1, 16)  OutScaling=2^0
  Add : Sum  OutDataType=fixdt(1, 16)  OutScaling=2^-10
  Cardiac inspiration : DiscretePulseGenerator  PulseType=Time based  Amplitude=1  Period=t_cardiac  PulseWidth=Cardiac_duty_cycle  PhaseDelay=0  SampleTime=1
  Constant : Constant  Value=0  OutDataType=fixdt(1, 16)  OutScaling=2^0
  From Workspace : FromWorkspace  VariableName=mdot_insp_am  SampleTime=0  Interpolate=off  OutputAfterFinalValue=Holding final value
  Insp flow (l/s)1 : Constant  Value=mdot_cardiac_am  OutDataType=sfix(16)  OutScaling=2^0
  Insp gas mixing : Subsystem
  Product1 : Product  OutDataType=sfix(16)  OutScaling=2^0  SaturateOnIntegerOverflow=on  RndMeth=Zero  InputSameDT=on  OutDataTypeStr=Inherit: Same as first input
  Product2 : Product  OutDataType=sfix(16)  OutScaling=2^0  SaturateOnIntegerOverflow=on  RndMeth=Zero  InputSameDT=on  OutDataTypeStr=Inherit: Same as first input
  Resp PWM : Subsystem
  Switch : Switch  Criteria=u2 ~= 0  OutDataType=fixdt(1, 16)  OutScaling=2^0
  To WS : ToWorkspace  VariableName=resp_timing  SampleTime=t_sample  SaveFormat=Array
  To WS1 : ToWorkspace  VariableName=mdot_insp  SampleTime=t_sample  SaveFormat=Array
  mdot insp total : Outport  OutDataType=sfix(16)  OutScaling=2^0
  Insp flow out : Outport  Port=2  OutDataType=sfix(16)  OutScaling=2^0
  tag scope: Resp_timing=global
  wires:
  From Workspace/1 -> Product1/1
  Insp gas mixing/1(Insp flow) -> Insp flow out/1
  Product1/1 -> Add/2
  Insp flow (l/s)1/1 -> Product2/1
  Add/1 -> mdot insp total/1, Insp gas mixing/1(mdot_insp), To WS1/1
  Switch/1 -> Add/1
  Product2/1 -> Switch/3
  Constant/1 -> Switch/1
  Cardiac inspiration/1 -> Product2/2
  Resp PWM/1(Out1) -> To WS/1, [Resp_timing], Product1/2, Switch/2
  O2/1 -> Insp gas mixing/2(O_2)
  CO2/1 -> Insp gas mixing/3(CO_2)
  N2/1 -> Insp gas mixing/4(N_2)

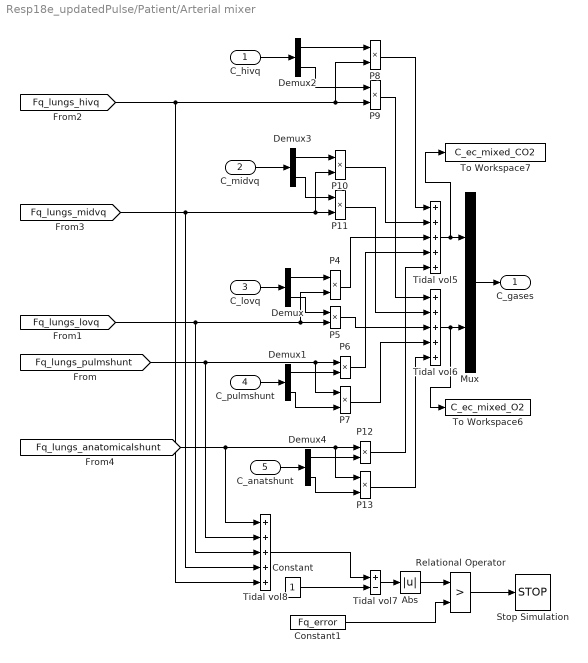
== system Resp18e_updatedPulse/Patient/Arterial mixer ==
  C_hivq : Inport  PortDimensions=2  OutDataType=sfix(16)  OutScaling=2^0
  C_midvq : Inport  Port=2  PortDimensions=2  OutDataType=sfix(16)  OutScaling=2^0
  C_lovq : Inport  Port=3  PortDimensions=2  OutDataType=sfix(16)  OutScaling=2^0
  C_pulmshunt : Inport  Port=4  PortDimensions=2  OutDataType=sfix(16)  OutScaling=2^0
  C_anatshunt : Inport  Port=5  PortDimensions=2  OutDataType=sfix(16)  OutScaling=2^0
  Abs : Abs  SaturateOnIntegerOverflow=on
  Constant : Constant  OutDataType=sfix(16)  OutScaling=2^0
  Constant1 : Constant  Value=Fq_error  OutDataType=sfix(16)  OutScaling=2^0
  Demux{,1..4} (5 alike) : Demux  Outputs=2
  Mux : Mux  Inputs=2
  P{4..13} (10 alike) : Product  Inputs=**  OutDataType=sfix(16)  OutScaling=2^0  SaturateOnIntegerOverflow=on  RndMeth=Zero  InputSameDT=on  OutDataTypeStr=Inherit: Same as first input
  Relational Operator : RelationalOperator  Operator=>  InputSameDT=on
  Stop Simulation : Stop
  Tidal vol5 : Sum  Inputs=+++++  OutDataType=sfix(16)  OutScaling=2^0  SaturateOnIntegerOverflow=on  InputSameDT=on  OutDataTypeStr=Inherit: Same as first input
  Tidal vol6 : Sum  Inputs=+++++  OutDataType=sfix(16)  OutScaling=2^0  SaturateOnIntegerOverflow=on  InputSameDT=on  OutDataTypeStr=Inherit: Same as first input
  Tidal vol7 : Sum  Inputs=+-  OutDataType=sfix(16)  OutScaling=2^0  SaturateOnIntegerOverflow=on  InputSameDT=on  OutDataTypeStr=Inherit: Same as first input
  Tidal vol8 : Sum  Inputs=+++++  OutDataType=sfix(16)  OutScaling=2^0  SaturateOnIntegerOverflow=on  InputSameDT=on  OutDataTypeStr=Inherit: Same as first input
  To Workspace6 : ToWorkspace  VariableName=C_ec_mixed_O2  SampleTime=t_sample  SaveFormat=Array
  To Workspace7 : ToWorkspace  VariableName=C_ec_mixed_CO2  SampleTime=t_sample  SaveFormat=Array
  C_gases : Outport  OutDataType=sfix(16)  OutScaling=2^0
  wires:
  Demux/2 -> P5/1
  Demux/1 -> P4/1
  Demux1/2 -> P7/2
  Demux1/1 -> P6/2
  C_pulmshunt/1 -> Demux1/1
  C_lovq/1 -> Demux/1
  Mux/1 -> C_gases/1
  Demux3/2 -> P11/1
  Demux3/1 -> P10/1
  C_midvq/1 -> Demux3/1
  Demux2/2 -> P9/1
  Demux2/1 -> P8/1
  C_hivq/1 -> Demux2/1
  P7/1 -> Tidal vol6/4
  P5/1 -> Tidal vol6/3
  P4/1 -> Tidal vol5/3
  P6/1 -> Tidal vol5/4
  P11/1 -> Tidal vol6/2
  P10/1 -> Tidal vol5/2
  P9/1 -> Tidal vol6/1
  P8/1 -> Tidal vol5/1
  Demux4/2 -> P13/2
  Demux4/1 -> P12/2
  C_anatshunt/1 -> Demux4/1
  P12/1 -> Tidal vol5/5
  P13/1 -> Tidal vol6/5
  Tidal vol6/1 -> Mux/2, To Workspace6/1
  Tidal vol5/1 -> Mux/1, To Workspace7/1
  [Fq_lungs_anatomicalshunt] -> P13/1, P12/1, Tidal vol8/1
  [Fq_lungs_pulmshunt] -> P7/1, P6/1, Tidal vol8/2
  [Fq_lungs_lovq] -> P5/2, P4/2, Tidal vol8/3
  [Fq_lungs_midvq] -> Tidal vol8/4, P11/2, P10/2
  [Fq_lungs_hivq] -> P9/2, P8/2, Tidal vol8/5
  Relational Operator/1 -> Stop Simulation/1
  Abs/1 -> Relational Operator/1
  Constant1/1 -> Relational Operator/2
  Constant/1 -> Tidal vol7/2
  Tidal vol7/1 -> Abs/1
  Tidal vol8/1 -> Tidal vol7/1

== system Resp18e_updatedPulse/Patient/Bag + exp measurements ==
  Inlet : Inport  OutDataType=sfix(16)  OutScaling=2^0
  CO2_exp : Integrator  InitialConditionSource=external
  Demux : Demux
  N2O_exp : Integrator  InitialConditionSource=external
  N2_exp : Integrator  InitialConditionSource=external
  O2_exp : Integrator  InitialConditionSource=external
  Term : Terminator
  Term3 : Terminator
  Tidal vol2 : Sum  Inputs=++++  OutDataType=sfix(16)  OutScaling=2^0  SaturateOnIntegerOverflow=on  InputSameDT=on  OutDataTypeStr=Inherit: Same as first input
  To WS6 : ToWorkspace  VariableName=mdot_CO2_exp  SampleTime=t_sample  SaveFormat=Array
  To Workspace10 : ToWorkspace  VariableName=mdot_exp_bag  SampleTime=t_sample  SaveFormat=Array
  To Workspace12 : ToWorkspace  VariableName=m_O2_exp  SampleTime=t_sample  SaveFormat=Array
  To Workspace9 : ToWorkspace  VariableName=m_CO2_exp  SampleTime=t_sample  SaveFormat=Array
  m_CO2_exp : Scope
      settings: YMin=0.3185  YMax=0.32175
  m_O2_exp : Scope
      settings: YMin=3.055  YMax=3.11  SaveName=ScopeData2
  mdot_CO2_exp : Scope
      settings: YMin=0  YMax=0.0007
  mdot_exp_bag : Scope
      settings: YMin=0  YMax=0.035  SaveName=ScopeData3
  zero : Constant  Value=0  OutDataType=sfix(16)  OutScaling=2^0
  wires:
  Inlet/1 -> Demux/1
  N2_exp/1 -> Term3/1
  O2_exp/1 -> To Workspace12/1, m_O2_exp/1
  N2O_exp/1 -> Term/1
  zero/1 -> N2O_exp/2, O2_exp/2, CO2_exp/2, N2_exp/2  "IC"
  Demux/4 -> N2_exp/1, Tidal vol2/1
  Demux/3 -> CO2_exp/1, To WS6/1, mdot_CO2_exp/1, Tidal vol2/2
  Demux/2 -> O2_exp/1, Tidal vol2/3
  Demux/1 -> N2O_exp/1, Tidal vol2/4
  Tidal vol2/1 -> To Workspace10/1, mdot_exp_bag/1
  CO2_exp/1 -> To Workspace9/1, m_CO2_exp/1

== system Resp18e_updatedPulse/Patient/Blood flow distribution control ==
  Pulmonary circulation : Subsystem
  Systemic circulation : Subsystem

== system Resp18e_updatedPulse/Patient/Brain ==
  In1 : Inport  OutDataType=sfix(16)  OutScaling=2^0
  Brain : Subsystem
  Delay_brain : Subsystem
  Out1 : Outport  OutDataType=sfix(16)  OutScaling=2^0
  wires:
  Brain/1(Cv_gases) -> Out1/1
  Delay_brain/1(Ca_gases_d) -> Brain/1(Ca_gases)
  In1/1 -> Delay_brain/1(C_gases)

== system Resp18e_updatedPulse/Patient/Cardiac mixing RV ==
  note: This block simlates mixing in the RV of the heart
      | and the Pulm artery
      | Ref: Lange et al JAP 21:1281 1966.
  Cmv_gases : Inport  PortDimensions=3  OutDataType=sfix(16)  OutScaling=2^0
  " " : Terminator
  "CO2 O2 " : Mux  Inputs=2
  CO2_RV : Integrator  InitialCondition=m_CO2_RV_b_i
  Demux : Demux  Outputs=3
  O2_RV : Integrator  InitialCondition=m_O2_RV_b_i
  P8 : Product  Inputs=**  OutDataType=sfix(16)  OutScaling=2^0  SaturateOnIntegerOverflow=on  RndMeth=Zero  InputSameDT=on  OutDataTypeStr=Inherit: Same as first input
  P9 : Product  Inputs=**  OutDataType=sfix(16)  OutScaling=2^0  SaturateOnIntegerOverflow=on  RndMeth=Zero  InputSameDT=on  OutDataTypeStr=Inherit: Same as first input
  RV_mixing : Gain  Gain=1/Vb_RV  ParameterDataType=sfix(16)  ParameterScaling=2^0  OutDataType=sfix(16)  OutScaling=2^0  SaturateOnIntegerOverflow=on  OutDataTypeStr=Inherit: Same as input  ParamDataTypeStr=Inherit: Same as input
  "RV_mixing " : Gain  Gain=1/Vb_RV  ParameterDataType=sfix(16)  ParameterScaling=2^0  OutDataType=sfix(16)  OutScaling=2^0  SaturateOnIntegerOverflow=on  OutDataTypeStr=Inherit: Same as input  ParamDataTypeStr=Inherit: Same as input
  Tidal vol4 : Sum  Inputs=-+  OutDataType=sfix(16)  OutScaling=2^0  SaturateOnIntegerOverflow=on  InputSameDT=on  OutDataTypeStr=Inherit: Same as first input
  Tidal vol5 : Sum  Inputs=+-  OutDataType=sfix(16)  OutScaling=2^0  SaturateOnIntegerOverflow=on  InputSameDT=on  OutDataTypeStr=Inherit: Same as first input
  Cv_gases : Outport  OutDataType=sfix(16)  OutScaling=2^0
  wires:
  "CO2 O2 "/1 -> Cv_gases/1
  Cmv_gases/1 -> Demux/1
  "RV_mixing "/1 -> "CO2 O2 "/2, Tidal vol5/2
  O2_RV/1 -> "RV_mixing "/1
  [Qpdot] -> P9/2, P8/2
  Tidal vol5/1 -> P9/1
  P9/1 -> O2_RV/1
  CO2_RV/1 -> RV_mixing/1
  P8/1 -> CO2_RV/1
  Tidal vol4/1 -> P8/1
  RV_mixing/1 -> "CO2 O2 "/1, Tidal vol4/1
  Demux/2 -> Tidal vol5/1
  Demux/1 -> Tidal vol4/2
  Demux/3 -> " "/1

== system Resp18e_updatedPulse/Patient/Cardiac o/p Control ==
  Qpdot : Constant  Value=Qpdot  OutDataType=sfix(16)  OutScaling=2^0
  tag scope: Qpdot=global
  wires:
  Qpdot/1 -> [Qpdot]  "Qpdot"

== system Resp18e_updatedPulse/Patient/Fat ==
  In1 : Inport  OutDataType=sfix(16)  OutScaling=2^0
  Delay_fat : Subsystem
  fat : Subsystem
  Out1 : Outport  OutDataType=sfix(16)  OutScaling=2^0
  wires:
  In1/1 -> Delay_fat/1(C_gases)
  Delay_fat/1(Ca_gases_d) -> fat/1(Ca_gases)
  fat/1(Cv_gases) -> Out1/1

== system Resp18e_updatedPulse/Patient/Heart ==
  In1 : Inport  OutDataType=sfix(16)  OutScaling=2^0
  Delay_heart : Subsystem
  Heart : Subsystem
  Out1 : Outport  OutDataType=sfix(16)  OutScaling=2^0
  wires:
  In1/1 -> Delay_heart/1(C_gases)
  Delay_heart/1(Ca_gases_d) -> Heart/1(Ca_gases)
  Heart/1(Cv_gases) -> Out1/1

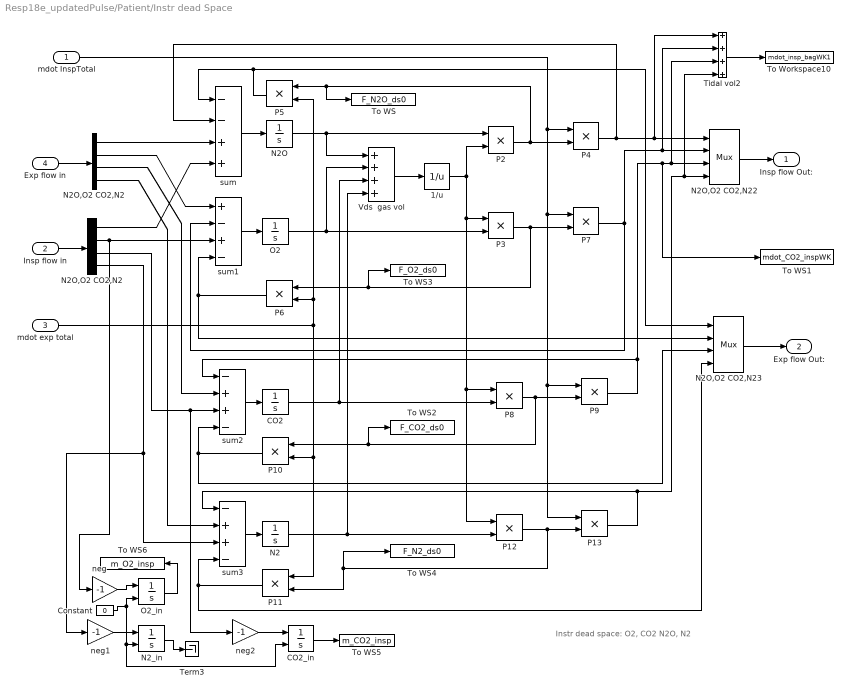
== system Resp18e_updatedPulse/Patient/Instr dead Space ==
  note: Instr dead space: O2, CO2 N2O, N2
  mdot InspTotal : Inport  PortDimensions=1  OutDataType=sfix(16)  OutScaling=2^0
  Insp flow in : Inport  Port=2  PortDimensions=4  OutDataType=sfix(16)  OutScaling=2^0
  mdot exp total : Inport  Port=3  PortDimensions=1  OutDataType=sfix(16)  OutScaling=2^0
  Exp flow in : Inport  Port=4  PortDimensions=4  OutDataType=sfix(16)  OutScaling=2^0
  1/u : Math  Operator=reciprocal  OutDataType=sfix(16)  OutScaling=2^0  SaturateOnIntegerOverflow=on
  CO2 : Integrator  InitialCondition=m_CO2_ds0_i
  CO2_in : Integrator  InitialConditionSource=external
  Constant : Constant  Value=0  OutDataType=sfix(16)  OutScaling=2^0
  N2 : Integrator  InitialCondition=m_N2_ds0_i
  N2O : Integrator  InitialCondition=m_N2O_ds0_i
  N2O,O2 CO2,N2 : Demux
  "N2O,O2 CO2,N2 " : Demux
  N2O,O2 CO2,N22 : Mux
  N2O,O2 CO2,N23 : Mux
  N2_in : Integrator  InitialConditionSource=external
  O2 : Integrator  InitialCondition=m_O2_ds0_i
  O2_in : Integrator  InitialConditionSource=external
  P{2..13} (12 alike) : Product  OutDataType=sfix(16)  OutScaling=2^0  SaturateOnIntegerOverflow=on  RndMeth=Zero  InputSameDT=on  OutDataTypeStr=Inherit: Same as first input
  Term3 : Terminator
  Tidal vol2 : Sum  Inputs=++++  OutDataType=sfix(16)  OutScaling=2^0  SaturateOnIntegerOverflow=on  InputSameDT=on  OutDataTypeStr=Inherit: Same as first input
  To WS : ToWorkspace  VariableName=F_N2O_ds0  SampleTime=t_sample  SaveFormat=Array
  To WS1 : ToWorkspace  VariableName=mdot_CO2_inspWK  SampleTime=t_sample  SaveFormat=Array
  To WS2 : ToWorkspace  VariableName=F_CO2_ds0  SampleTime=t_sample  SaveFormat=Array
  To WS3 : ToWorkspace  VariableName=F_O2_ds0  SampleTime=t_sample  SaveFormat=Array
  To WS4 : ToWorkspace  VariableName=F_N2_ds0  SampleTime=t_sample  SaveFormat=Array
  To WS5 : ToWorkspace  VariableName=m_CO2_insp  SampleTime=t_sample  SaveFormat=Array
  To WS6 : ToWorkspace  VariableName=m_O2_insp  SampleTime=t_sample  SaveFormat=Array
  To Workspace10 : ToWorkspace  VariableName=mdot_insp_bagWK1  SampleTime=t_sample  SaveFormat=Array
  Vds  gas vol : Sum  Inputs=++++  OutDataType=sfix(16)  OutScaling=2^0  SaturateOnIntegerOverflow=on  InputSameDT=on  OutDataTypeStr=Inherit: Same as first input
  neg : Gain  Gain=-1  ParameterDataType=sfix(16)  ParameterScaling=2^0  OutDataType=sfix(16)  OutScaling=2^0  SaturateOnIntegerOverflow=on  OutDataTypeStr=Inherit: Same as input  ParamDataTypeStr=Inherit: Same as input
  neg1 : Gain  Gain=-1  ParameterDataType=sfix(16)  ParameterScaling=2^0  OutDataType=sfix(16)  OutScaling=2^0  SaturateOnIntegerOverflow=on  OutDataTypeStr=Inherit: Same as input  ParamDataTypeStr=Inherit: Same as input
  neg2 : Gain  Gain=-1  ParameterDataType=sfix(16)  ParameterScaling=2^0  OutDataType=sfix(16)  OutScaling=2^0  SaturateOnIntegerOverflow=on  OutDataTypeStr=Inherit: Same as input  ParamDataTypeStr=Inherit: Same as input
  sum : Sum  Inputs=--++  OutDataType=sfix(16)  OutScaling=2^0  SaturateOnIntegerOverflow=on  InputSameDT=on  OutDataTypeStr=Inherit: Same as first input
  sum1 : Sum  Inputs=+-+-  OutDataType=sfix(16)  OutScaling=2^0  SaturateOnIntegerOverflow=on  InputSameDT=on  OutDataTypeStr=Inherit: Same as first input
  sum2 : Sum  Inputs=-++-  OutDataType=sfix(16)  OutScaling=2^0  SaturateOnIntegerOverflow=on  InputSameDT=on  OutDataTypeStr=Inherit: Same as first input
  sum3 : Sum  Inputs=-++-  OutDataType=sfix(16)  OutScaling=2^0  SaturateOnIntegerOverflow=on  InputSameDT=on  OutDataTypeStr=Inherit: Same as first input
  Insp flow Out: : Outport  OutDataType=sfix(16)  OutScaling=2^0
  Exp flow Out: : Outport  Port=2  OutDataType=sfix(16)  OutScaling=2^0
  wires:
  N2/1 -> Vds  gas vol/4, P12/2
  P11/1 -> N2O,O2 CO2,N23/4, sum3/4
  P3/1 -> P7/2, To WS3/1, P6/1
  P13/1 -> sum3/1, N2O,O2 CO2,N22/4, Tidal vol2/4
  N2O,O2 CO2,N2/4 -> sum3/2
  P12/1 -> P13/2, P11/2, To WS4/1
  sum3/1 -> N2/1
  N2O,O2 CO2,N2/3 -> sum2/2
  P9/1 -> sum2/1, N2O,O2 CO2,N22/3, Tidal vol2/3, To WS1/1
  N2O,O2 CO2,N2/1 -> sum/3
  P4/1 -> sum/2, N2O,O2 CO2,N22/1, Tidal vol2/1
  "N2O,O2 CO2,N2 "/1 -> sum/4
  Insp flow in/1 -> "N2O,O2 CO2,N2 "/1
  N2O,O2 CO2,N2/2 -> sum1/1
  Exp flow in/1 -> N2O,O2 CO2,N2/1
  N2O,O2 CO2,N22/1 -> Insp flow Out:/1
  N2O,O2 CO2,N23/1 -> Exp flow Out:/1
  P10/1 -> sum2/4, N2O,O2 CO2,N23/3
  mdot exp total/1 -> P11/1, P10/2, P5/2, P6/2
  P8/1 -> P9/2, To WS2/1, P10/1
  CO2/1 -> P8/2, Vds  gas vol/3
  P2/1 -> P5/1, To WS/1, P4/2
  sum2/1 -> CO2/1
  mdot InspTotal/1 -> P7/1, P13/1, P9/1, P4/1
  sum/1 -> N2O/1
  sum1/1 -> O2/1
  Vds  gas vol/1 -> 1/u/1
  1/u/1 -> P12/1, P8/1, P3/1, P2/2
  P7/1 -> sum1/2, N2O,O2 CO2,N22/2, Tidal vol2/2
  N2O/1 -> P2/1, Vds  gas vol/1
  O2/1 -> P3/2, Vds  gas vol/2
  P6/1 -> N2O,O2 CO2,N23/2, sum1/4
  P5/1 -> N2O,O2 CO2,N23/1, sum/1
  "N2O,O2 CO2,N2 "/2 -> neg/1, sum1/3
  neg/1 -> O2_in/1
  N2_in/1 -> Term3/1
  neg1/1 -> N2_in/1
  "N2O,O2 CO2,N2 "/4 -> sum3/3, neg1/1
  Constant/1 -> O2_in/2, N2_in/2, CO2_in/2
  neg2/1 -> CO2_in/1
  "N2O,O2 CO2,N2 "/3 -> sum2/3, neg2/1
  CO2_in/1 -> To WS5/1
  O2_in/1 -> To WS6/1
  Tidal vol2/1 -> To Workspace10/1

== system Resp18e_updatedPulse/Patient/Kidneys ==
  In1 : Inport  OutDataType=sfix(16)  OutScaling=2^0
  Delay_kidneys : Subsystem
  Kidneys : Subsystem
  Out1 : Outport  OutDataType=sfix(16)  OutScaling=2^0
  wires:
  Kidneys/1(Cv_gases) -> Out1/1
  Delay_kidneys/1(Ca_gases_d) -> Kidneys/1(Ca_gases)
  In1/1 -> Delay_kidneys/1(C_gases)

== system Resp18e_updatedPulse/Patient/LV + Aorta ==
  In1 : Inport  OutDataType=sfix(16)  OutScaling=2^0
  Arterial blood gas measurements : Subsystem
  Cardiac mixing LV : Subsystem
  Delay_common : Subsystem
  Out1 : Outport  OutDataType=sfix(16)  OutScaling=2^0
  wires:
  Cardiac mixing LV/1(Ca_gases) -> Arterial blood gas measurements/1(C_a_gases), Delay_common/1(C_gases)
  Delay_common/1(Ca_gases_d) -> Out1/1
  In1/1 -> Cardiac mixing LV/1(Cec_gases)

== system Resp18e_updatedPulse/Patient/Large Veins ==
  Heart : Inport  OutDataType=sfix(16)  OutScaling=2^0
  Brain : Inport  Port=2  OutDataType=sfix(16)  OutScaling=2^0
  Per shunt : Inport  Port=3  OutDataType=sfix(16)  OutScaling=2^0
  Liver_gut : Inport  Port=4  OutDataType=sfix(16)  OutScaling=2^0
  Kidneys : Inport  Port=5  OutDataType=sfix(16)  OutScaling=2^0
  Muscle : Inport  Port=6  OutDataType=sfix(16)  OutScaling=2^0
  Lean : Inport  Port=7  OutDataType=sfix(16)  OutScaling=2^0
  Fat : Inport  Port=8  OutDataType=sfix(16)  OutScaling=2^0
  Flow prop mix : Subsystem
  Flow prop mix1 : Subsystem
  Flow prop mix2 : Subsystem
  Flow prop mix3 : Subsystem
  Flow prop mix4 : Subsystem
  Flow prop mix5 : Subsystem
  Flow prop mixer2 : Subsystem
  Mixed venous measurements : Subsystem
  Mixed Venous : Outport  OutDataType=sfix(16)  OutScaling=2^0
  wires:
  Flow prop mix/1(C_gases) -> Flow prop mixer2/2(C2_gases)
  Flow prop mix1/1(C_gases) -> Flow prop mix/2(C2_gases)
  Flow prop mix2/1(C_gases) -> Flow prop mix1/2(C2_gases)
  Flow prop mix4/1(C_gases) -> Flow prop mix2/2(C2_gases)
  Flow prop mixer2/1(C_gases) -> Flow prop mix5/2(C2_gases)
  Flow prop mix5/1(C_gases) -> Flow prop mix3/1(C1_gases)
  Heart/1 -> Flow prop mix3/2(C2_gases)
  Brain/1 -> Flow prop mix5/1(C1_gases)
  Per shunt/1 -> Flow prop mixer2/1(C1_gases)
  Liver_gut/1 -> Flow prop mix/1(C1_gases)
  Kidneys/1 -> Flow prop mix1/1(C1_gases)
  Muscle/1 -> Flow prop mix2/1(C1_gases)
  Lean/1 -> Flow prop mix4/1(C1_gases)
  Fat/1 -> Flow prop mix4/2(C2_gases)
  Flow prop mix3/1(C_gases) -> Mixed Venous/1, Mixed venous measurements/1(Cmv_gases)

== system Resp18e_updatedPulse/Patient/Liver & gut ==
  In1 : Inport  OutDataType=sfix(16)  OutScaling=2^0
  Delay_hepatic : Subsystem
  Delay_portal : Subsystem
  Flow prop mixer : Subsystem
  Liver : Subsystem
  Portal : Subsystem
  Out1 : Outport  OutDataType=sfix(16)  OutScaling=2^0
  wires:
  Liver/1(Cv_gases) -> Out1/1
  In1/1 -> Delay_hepatic/1(C_gases), Delay_portal/1(C_gases)
  Delay_hepatic/1(Ca_gases_d) -> Flow prop mixer/1(C1_gases)
  Flow prop mixer/1(C_gases) -> Liver/1(Ca_gases)
  Delay_portal/1(Ca_gases_d) -> Portal/1(Ca_gases)
  Portal/1(Cv_gases) -> Flow prop mixer/2(C2_gases)

== system Resp18e_updatedPulse/Patient/Lung tissue alvds ==
  note: This block calculates:
      | 1. Alveolar partial pressures of CO2 & O2
      | 2. CO2 uptake by lung tissues
      | 3. CO2 uptake by pulmonary capillaries
      | 4. O2 uptake by pulmonary capillaries
  note: Alveolar deadspace has lng tissue exchanging CO2 with gas compartment.
      | No exchange with pulmonary blood
  FA_gases : Inport  PortDimensions=2  OutDataType=sfix(16)  OutScaling=2^0
  CO2 O2 : Mux  Inputs=2
  Demux : Demux  Outputs=2
  Lung tissue : Subsystem  Description=Calculates quantity of CO2 stored in two lung tissue compartments (fast & slow)
  O2 : Constant  Value=0  OutDataType=sfix(16)  OutScaling=2^0
  P3 : Product  Inputs=**  OutDataType=sfix(16)  OutScaling=2^0  SaturateOnIntegerOverflow=on  RndMeth=Zero  InputSameDT=on  OutDataTypeStr=Inherit: Same as first input
  P4 : Product  Inputs=**  OutDataType=sfix(16)  OutScaling=2^0  SaturateOnIntegerOverflow=on  RndMeth=Zero  InputSameDT=on  OutDataTypeStr=Inherit: Same as first input
  To Workspace8 : ToWorkspace  VariableName=P_A_CO2_alvds  SampleTime=t_sample  SaveFormat=Array
  To Workspace9 : ToWorkspace  VariableName=P_A_O2_alvds  SampleTime=t_sample  SaveFormat=Array
  sum3 : Sum  Inputs=++-  OutDataType=sfix(16)  OutScaling=2^0  SaturateOnIntegerOverflow=on  InputSameDT=on  OutDataTypeStr=Inherit: Same as first input
  mdot_gases : Outport  OutDataType=sfix(16)  OutScaling=2^0
  wires:
  [P_baro] -> sum3/1
  [P_A_H2O] -> sum3/3
  FA_gases/1 -> Demux/1
  [P_alv] -> sum3/2
  Demux/1 -> P3/1
  Demux/2 -> P4/1
  sum3/1 -> P4/2, P3/2
  P4/1 -> To Workspace9/1  "PA_O2"
  P3/1 -> To Workspace8/1, Lung tissue/1(PA_CO2)  "PA_CO2"
  Lung tissue/1(mdot_CO2_tissue) -> CO2 O2/1
  O2/1 -> CO2 O2/2
  CO2 O2/1 -> mdot_gases/1

== system Resp18e_updatedPulse/Patient/Misc values ==
  Qpdot : Constant  Value=P_A_H2O  OutDataType=sfix(16)  OutScaling=2^0
  Qpdot1 : Constant  Value=P_baro  OutDataType=sfix(16)  OutScaling=2^0
  tag scope: P_A_H2O=global, P_baro=global
  wires:
  Qpdot/1 -> [P_A_H2O]
  Qpdot1/1 -> [P_baro]

== system Resp18e_updatedPulse/Patient/Muscle ==
  In1 : Inport  OutDataType=sfix(16)  OutScaling=2^0
  Delay_muscle : Subsystem
  Muscle : Subsystem
  Out1 : Outport  OutDataType=sfix(16)  OutScaling=2^0
  wires:
  In1/1 -> Delay_muscle/1(C_gases)
  Delay_muscle/1(Ca_gases_d) -> Muscle/1(Ca_gases)
  Muscle/1(Cv_gases) -> Out1/1

== system Resp18e_updatedPulse/Patient/Other lean ==
  In1 : Inport  OutDataType=sfix(16)  OutScaling=2^0
  Delay_lean : Subsystem
  Lean : Subsystem
  Out1 : Outport  OutDataType=sfix(16)  OutScaling=2^0
  wires:
  Lean/1(Cv_gases) -> Out1/1
  Delay_lean/1(Ca_gases_d) -> Lean/1(Ca_gases)
  In1/1 -> Delay_lean/1(C_gases)

== system Resp18e_updatedPulse/Patient/Periph Shunt ==
  In1 : Inport  OutDataType=sfix(16)  OutScaling=2^0
  Delay_pershunt : Subsystem
  Out1 : Outport  OutDataType=sfix(16)  OutScaling=2^0
  wires:
  In1/1 -> Delay_pershunt/1(C_gases)
  Delay_pershunt/1(Ca_gases_d) -> Out1/1

== system Resp18e_updatedPulse/Patient/Pulm Cap gas transfer ==
  note: Calculates total accumulated CO2 +O2 transfer between
      | alveolar compartments and pulmonary capillaries
      | Label starts with m so that this integrator does not affect
      | O2 & CO2 mass balance calcs
  Constant : Constant  Value=0  OutDataType=sfix(16)  OutScaling=2^0
  Constant1 : Constant  Value=0  OutDataType=sfix(16)  OutScaling=2^0
  To WS5 : ToWorkspace  VariableName=m_CO2_a_A  SampleTime=t_sample  SaveFormat=Array
  To WS6 : ToWorkspace  VariableName=m_O2_a_A  SampleTime=t_sample  SaveFormat=Array
  m_CO2_a_A : Integrator  InitialConditionSource=external
  m_O2_a_A : Integrator  InitialConditionSource=external
  sum1 : Sum  Inputs=+++  OutDataType=sfix(16)  OutScaling=2^0  SaturateOnIntegerOverflow=on  InputSameDT=on  OutDataTypeStr=Inherit: Same as first input
  sum2 : Sum  Inputs=+++  OutDataType=sfix(16)  OutScaling=2^0  SaturateOnIntegerOverflow=on  InputSameDT=on  OutDataTypeStr=Inherit: Same as first input
  wires:
  m_CO2_a_A/1 -> To WS5/1
  Constant/1 -> m_CO2_a_A/2
  sum1/1 -> m_CO2_a_A/1
  [mdot_CO2_a_A_hivq] -> sum1/1
  [mdot_CO2_a_A_midvq] -> sum1/2
  [mdot_CO2_a_A_lovq] -> sum1/3
  m_O2_a_A/1 -> To WS6/1
  Constant1/1 -> m_O2_a_A/2
  sum2/1 -> m_O2_a_A/1
  [mdot_O2_a_A_hivq] -> sum2/1
  [mdot_O2_a_A_midvq] -> sum2/2
  [mdot_O2_a_A_lovq] -> sum2/3
